simulink model "PLL_with_3GHz_VCO"  (R2022a)
settings: Solver=VariableStepAuto  StartTime=0.0  StopTime=15e-06  RelTol=1e-3
model workspace (MAT data in the model file):
  Frequency_6 = 3200000000.02
  LockTime_6 = 1.1675e-06
  PnFrequencyOffset_6 = [100000 1000000 3000000 10000000]
  TargetFrequency_6 = 3210000000
  TargetLockTime_6 = 3e-06
  TargetPhaseNoise_6 = [-108 -134 -145 -154]
  uniqueStringPll_6 = '14_1886'
  uniqueString_6 = '81_4724'
libraries: dspswit3 x1, msbPllArchitectures x1, msbPllMeasurements x1
settings Model: Creator=The MathWorks, Inc.  LastModifiedBy=rollo
settings SolverCC: AlgebraicLoopSolver=TrustRegion
settings DebuggingCC: UnconnectedInputMsg=warning  UnconnectedOutputMsg=warning  UnconnectedLineMsg=warning  SFMachineParentedDataDiag=warning
settings RTWCC: DLArmComputeVersion=19.05

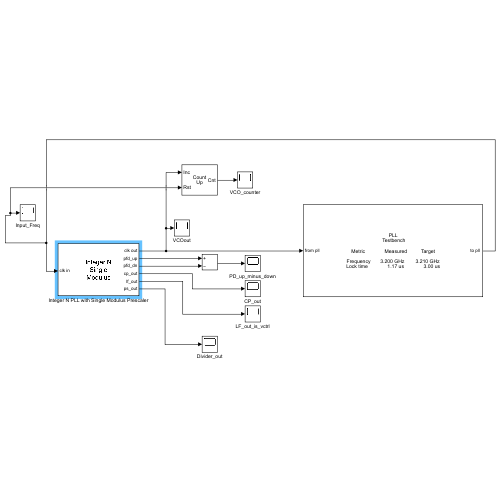
[thumbnail: Simulink's stored preview of the top-level diagram]
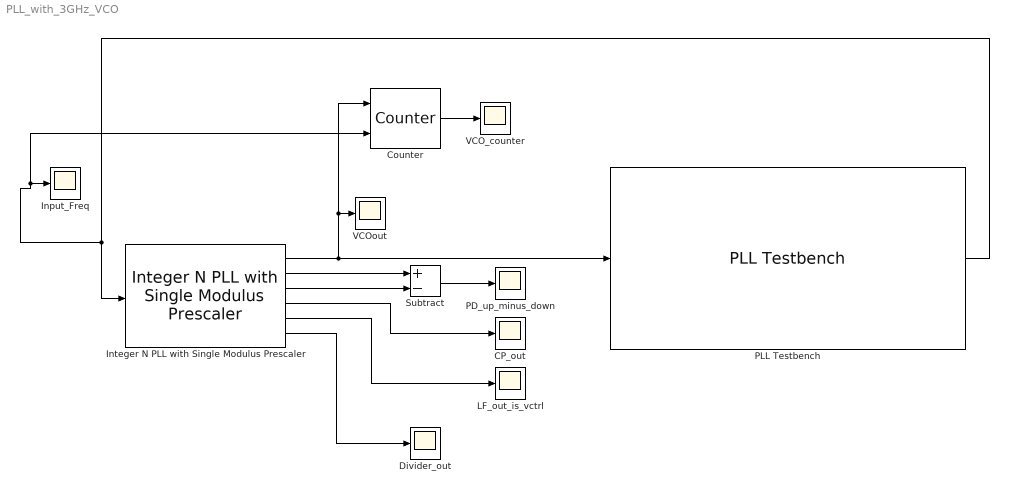
== system PLL_with_3GHz_VCO ==
  CP_out : Scope
  Counter : dspswit3/Counter  Direction=Up  CountEvent=Rising edge  CounterSize=User defined  MaxCount=255  InitialCount=0  Output=Count  HitValue=32  ResetInput=on  SamplesPerFrame=1  Ts=1  CntDtype=double  HitDtype=Logical
  Divider_out : Scope
  Input_Freq : Scope
  Integer N PLL with Single Modulus Prescaler : msbPllArchitectures/Integer N PLL with Single Modulus Prescaler  DeadbandCompensation=30e-12  EnableImpairments=off  DefaultOrAdvanced=Default  MaxFreqInterest=10e9  RiseFallTime=30e-12  PropDelay=50e-12  OutputCurrent=0.02e-3  InputThreshold=0.5  EnableCurrentImpairments=off  CurrentImbalance=1e-7  LeakageCurrent=1e-8  EnableTimingImpairments=off  DefaultOrAdvancedCp=Default  MaxFreqInterestCp=10e9  RiseFallUp=50e-12  PropDelayUp=60e-12  RiseFallDown=20e-12  PropDelayDown=40e-12  SpecifyUsing=Output frequency vs. control voltage  Kvco=9.49e9  ControlVoltage="[-0.2\t-0.1\t0\t0.0999999999999999\t0.2\t0.9]"  OutputFrequency=|  MaxKvco=16799640000  Fo=3.21e9  Amplitude=1  AddPhaseNoise=off  Foffset=[100e3 1e6 3e6 10e6]  PhaseNoise=[-108 -134 -145 -154]  N=128  Nmin=128  CompSelectionMethod=Manual  Fc=160e3  Phi=45  FilterType=2nd order passive  C1=94e-15  C2=940e-15  C3=10e-15  C4=331.5752  R2=30e3  R3=1e3  R4=28.1695  LfEnableImpairments=off  Temperature=30  pfd_up_dn=on  cp_out=on  lf_out=on  ps_out=on  ol_opt=on  cl_opt=on  ExtraBuffer=off  NBufferFilter=1000  NBuffer=10
      | [
      | 942.036E+06	2.622E+09	3.258E+09	3.511E+09	3.613E+09	3.717E+09
      | ]
      settings: SourceProductBaseCode=AM
  LF_out_is_vctrl : Scope
  PD_up_minus_down : Scope
  PLL Testbench : msbPllMeasurements/PLL Testbench  InputAmplitude=1  ClkFreq=25e6  FrequencyMeasureOption=on  CurrentFrequency=0  LockTimeOption=on  ExpectedFreq=3.21e9  FreqErrorTol=0.1e9  CurrentLockTime=0  PhaseNoiseOption=off  SampleRate=8*2.8e9  ResBandwidth=50e3  SpectralAverages=4  HoldOffTime=1.5e-5  PhaseNoiseFreqOffset=[100e3 1e6 3e6 10e6]  OpenSpectrum=off  ExtraBuffer=off  NBuffer=10  PowerVector=0  FrequencyVector=0  TargetFreq=2.1e9  TargetLockTime=3e-6  TargetPhaseNoiseVector=[-108 -134 -145 -154]
      settings: SourceProductBaseCode=AM  SignalType=Square
  Subtract : Sum  Inputs=+-
  VCO_counter : Scope
  VCOout : Scope
  wires:
  PLL Testbench/1 -> Counter/2, Input_Freq/1, Integer N PLL with Single Modulus Prescaler/1
  Integer N PLL with Single Modulus Prescaler/1 -> Counter/1, VCOout/1, PLL Testbench/1
  Integer N PLL with Single Modulus Prescaler/5 -> LF_out_is_vctrl/1
  Integer N PLL with Single Modulus Prescaler/2 -> Subtract/1
  Integer N PLL with Single Modulus Prescaler/3 -> Subtract/2
  Subtract/1 -> PD_up_minus_down/1
  Integer N PLL with Single Modulus Prescaler/4 -> CP_out/1
  Integer N PLL with Single Modulus Prescaler/6 -> Divider_out/1
  Counter/1 -> VCO_counter/1
